simulink model "trail2"  (R2020b)
settings: Solver=FixedStepAuto  StartTime=0.0  StopTime=60  FixedStep=10  RelTol=1e-3
libraries: simulink x2
settings Model: Creator=99003785  LastModifiedBy=99003785

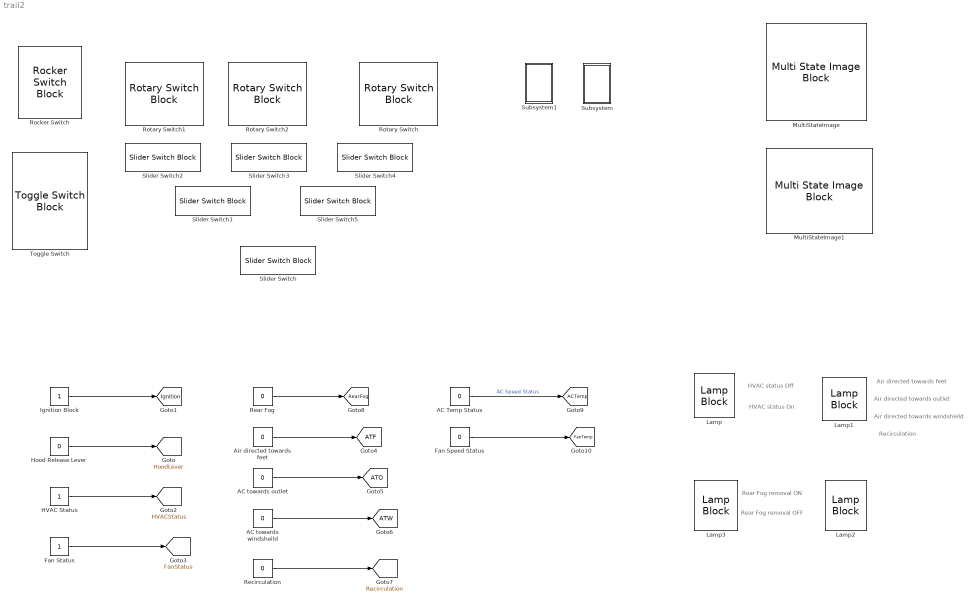
== system trail2 ==
  note: Rear Fog removal OFF
  note: Recirculation
  note: Air directed towards feet
  note: Air directed towards outlet
  note: Air directed towards windshield
  note: HVAC status On
  note: Rear Fog removal ON
  note: HVAC status Off
  AC Temp Status : Constant  Value=0
  AC towards outlet : Constant  Value=0
  AC towards windsheild : Constant  Value=0
  Air directed towards feet : Constant  Value=0
  Fan Speed Status : Constant  Value=0
  Fan Status : Constant
  HVAC Status : Constant
  Hood Release Lever : Constant  Value=0
  Ignition Block : Constant
  Lamp{,1..3} (4 alike) : LampBlock
  MultiStateImage : MultiStateImageBlock
  MultiStateImage1 : MultiStateImageBlock
  Rear Fog : Constant  Value=0
  Recirculation : Constant  Value=0
  Rocker Switch : RockerSwitchBlock
      settings: Values={{'On', 'Off'}, [1 0]}
  Rotary Switch : RotarySwitchBlock
      settings: Values={{'Off', 'Low', 'Medium', 'High'}, [0 1 2 3]}
  Rotary Switch1 : RotarySwitchBlock
      settings: Values={{'Off', 'Low', 'Medium', 'High'}, [0 1 2 3]}
  Rotary Switch2 : RotarySwitchBlock
      settings: Values={{'Off', 'AC', 'Heater', 'Air-Vent'}, [0 1 2 3]}
  Slider Switch{,1..5} (6 alike) : SliderSwitchBlock
      settings: Values={{'Off', 'On'}, [0 1]}
  Subsystem : Subsystem
  Subsystem1 : Subsystem
  Toggle Switch : ToggleSwitchBlock
      settings: Values={{'Off', 'On'}, [0 1]}
  tag scope: ACTemp=global, ATF=global, ATO=global, ATW=global, FanStatus=global, FanTemp=global, HVACStatus=global, HoodLever=global, Ignition=global, RearFog=global, Recirculation=global
  wires:
  Hood Release Lever/1 -> [HoodLever]
  Ignition Block/1 -> [Ignition]
  HVAC Status/1 -> [HVACStatus]
  Fan Status/1 -> [FanStatus]
  Air directed towards feet/1 -> [ATF]
  AC towards outlet/1 -> [ATO]
  Rear Fog/1 -> [RearFog]
  Recirculation/1 -> [Recirculation]
  AC towards windsheild/1 -> [ATW]
  AC Temp Status/1 -> [ACTemp]  "AC Speed Status"
  Fan Speed Status/1 -> [FanTemp]

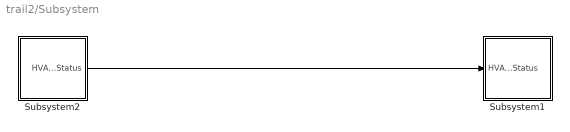
== system trail2/Subsystem ==
  Subsystem1 : Subsystem
  Subsystem2 : Subsystem
  wires:
  Subsystem2/1(HVAC Status) -> Subsystem1/1(HVAC Status)

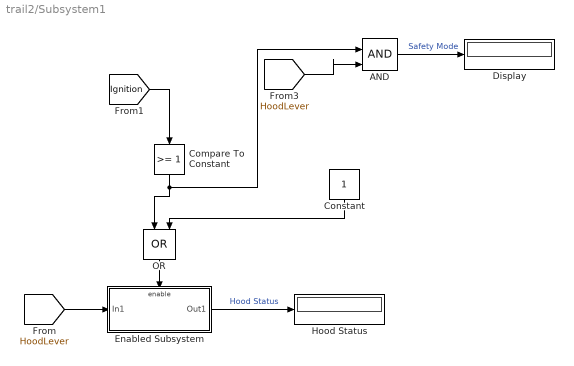
== system trail2/Subsystem1 ==
  AND : Logic  IconShape=distinctive  AllPortsSameDT=off  OutDataTypeStr=boolean
  Compare To Constant : simulink/Logic and Bit Operations/Compare To Constant  relop=>=  const=1  OutDataTypeStr=boolean
  Constant : Constant
  Display : Display
  Enabled Subsystem : Subsystem  TreatAsAtomicUnit=on
  Hood Status : Display
  OR : Logic  Operator=OR  IconShape=distinctive  AllPortsSameDT=off  OutDataTypeStr=boolean
  wires:
  AND/1 -> Display/1  "Safety Mode"
  OR/1 -> Enabled Subsystem/Enable
  Compare To Constant/1 -> AND/1, OR/1
  Constant/1 -> OR/2
  [Ignition] -> Compare To Constant/1
  Enabled Subsystem/1(Out1) -> Hood Status/1  "Hood Status"
  [HoodLever] -> Enabled Subsystem/1(In1)
  [HoodLever] -> AND/2

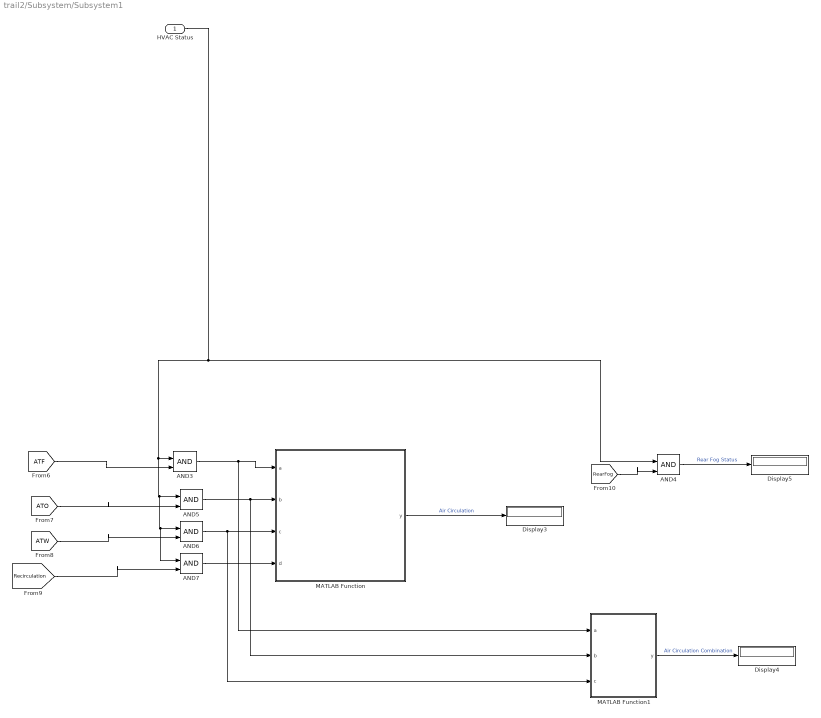
== system trail2/Subsystem/Subsystem1 ==
  HVAC Status : Inport
  AND{3..7} (5 alike) : Logic  IconShape=distinctive  AllPortsSameDT=off  OutDataTypeStr=boolean
  Display3 : Display
  Display4 : Display
  Display5 : Display
  MATLAB Function : MATLAB Function  TreatAsAtomicUnit=on
  MATLAB Function1 : MATLAB Function  TreatAsAtomicUnit=on
  wires:
  AND3/1 -> MATLAB Function1/1(a), MATLAB Function/1(a)
  AND4/1 -> Display5/1  "Rear Fog Status"
  AND6/1 -> MATLAB Function1/3(c), MATLAB Function/3(c)
  AND5/1 -> MATLAB Function1/2(b), MATLAB Function/2(b)
  MATLAB Function1/1(y) -> Display4/1  "Air Circulation Combination"
  AND7/1 -> MATLAB Function/4(d)
  [ATW] -> AND6/2
  [RearFog] -> AND4/2
  [ATO] -> AND5/2
  HVAC Status/1 -> AND7/1, AND6/1, AND5/1, AND3/1, AND4/1
  MATLAB Function/1(y) -> Display3/1  "Air Circulation"
  [Recirculation] -> AND7/2
  [ATF] -> AND3/2

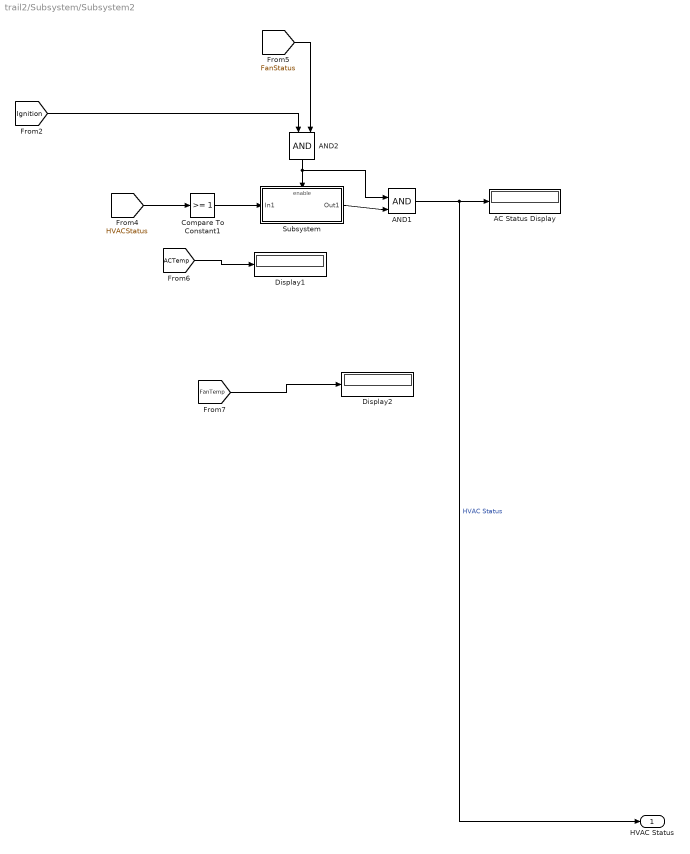
== system trail2/Subsystem/Subsystem2 ==
  AC Status Display : Display
  AND1 : Logic  IconShape=distinctive  AllPortsSameDT=off  OutDataTypeStr=boolean
  AND2 : Logic  IconShape=distinctive  AllPortsSameDT=off  OutDataTypeStr=boolean
  Compare To Constant1 : simulink/Logic and Bit Operations/Compare To Constant  relop=>=  const=1  OutDataTypeStr=boolean
  Display1 : Display
  Display2 : Display
  Subsystem : Subsystem
  HVAC Status : Outport
  wires:
  [FanTemp] -> Display2/1
  [Ignition] -> AND2/1
  AND1/1 -> HVAC Status/1, AC Status Display/1  "HVAC Status"
  [HVACStatus] -> Compare To Constant1/1
  [ACTemp] -> Display1/1
  [FanStatus] -> AND2/2
  Compare To Constant1/1 -> Subsystem/1(In1)
  AND2/1 -> AND1/1, Subsystem/Enable
  Subsystem/1(Out1) -> AND1/2

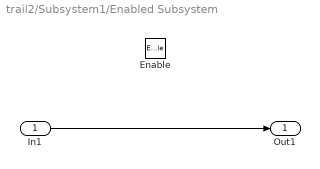
== system trail2/Subsystem1/Enabled Subsystem ==
  In1 : Inport
  Enable : EnablePort
  Out1 : Outport  InitialOutput=0  VectorParamsAs1DForOutWhenUnconnected=off
  wires:
  In1/1 -> Out1/1

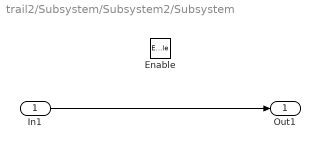
== system trail2/Subsystem/Subsystem2/Subsystem ==
  In1 : Inport
  Enable : EnablePort
  Out1 : Outport
  wires:
  In1/1 -> Out1/1

== matlab function trail2/Subsystem/Subsystem1/MATLAB Function1 ==
  data: a input; b input; c input; y output
function y = fcn(a,b,c)
    if a==1&& b==1 && c==1
        y=1;
    elseif a==1 && b==1 && c==0
        y=2;
    elseif a==1 && b==0 && c==1
        y=3;
    elseif a==0 && b==1 && c==1
        y=4;
    else
        y=0;
    end

end

== matlab function trail2/Subsystem/Subsystem1/MATLAB Function ==
  data: a input; b input; y output; c input; d input
function y = fcn(a, b, c, d)
    if a==1 && b==0 && c==0 && d==0
        y=1;
    elseif a==0 && b==1 &&c==0 && d==0
        y=2;
    elseif a==0 && b==0 &&c==1 && d==0
        y=3;
    elseif a==0 && b==0 &&c==0 && d==1
        y=4;
    else
        y=0;
    end
    

end
